simulink model "model3_bode"  (R2022a)
settings: Solver=VariableStepAuto  StartTime=0.0  StopTime=10.0  RelTol=1e-3
undefined symbols (not defined in the file or in its folder): car, disturb, E2TD, E2TN, T2VD
settings Model: Creator=Jirapu  LastModifiedBy=Jirapu

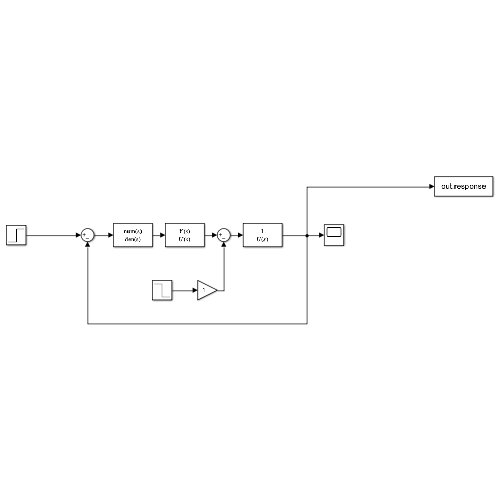
[thumbnail: Simulink's stored preview of the top-level diagram]
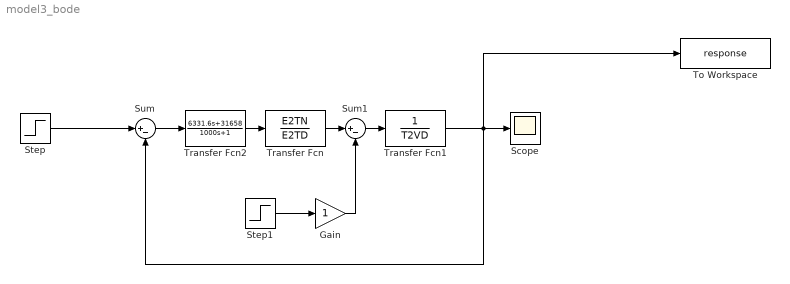
== system model3_bode ==
  Gain : Gain
  Scope : Scope
  Step : Step  Time=0  After=car.V_desire  SampleTime=0
  Step1 : Step  Time=0  After=disturb  SampleTime=0
  Sum : Sum  Inputs=|+-
  Sum1 : Sum  Inputs=|+-
  To Workspace : ToWorkspace  VariableName=response  SaveFormat=Timeseries  SampleTime=-1
  Transfer Fcn : TransferFcn  Numerator=E2TN  Denominator=E2TD
  Transfer Fcn1 : TransferFcn  Denominator=T2VD
  Transfer Fcn2 : TransferFcn  Numerator=[6331.6 31658]  Denominator=[1000 1]
  wires:
  Transfer Fcn1/1 -> To Workspace/1, Sum/2, Scope/1
  Step1/1 -> Gain/1
  Transfer Fcn/1 -> Sum1/1
  Step/1 -> Sum/1
  Gain/1 -> Sum1/2
  Sum1/1 -> Transfer Fcn1/1
  Transfer Fcn2/1 -> Transfer Fcn/1
  Sum/1 -> Transfer Fcn2/1
